simulink model "PID4"  (R2021a)
settings: Solver=VariableStepAuto  StartTime=0.0  StopTime=100  RelTol=1e-3
settings Model: Creator=Office  LastModifiedBy=Office

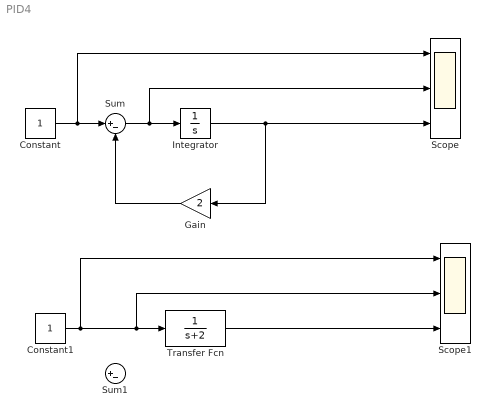
== system PID4 ==
  Constant : Constant
  Constant1 : Constant
  Gain : Gain  Gain=2
  Integrator : Integrator
  Scope : Scope  NumInputPorts=3
  Scope1 : Scope  NumInputPorts=3
  Sum : Sum  Inputs=|+-
  Sum1 : Sum  Inputs=|+-
  Transfer Fcn : TransferFcn  Denominator=[1 2]
  wires:
  Integrator/1 -> Gain/1, Scope/3
  Constant/1 -> Scope/1, Sum/1
  Gain/1 -> Sum/2
  Sum/1 -> Scope/2, Integrator/1
  Transfer Fcn/1 -> Scope1/3
  Constant1/1 -> Scope1/2, Transfer Fcn/1, Scope1/1
